simulink model "batterworth_test"  (R2021b)
settings: Solver=VariableStepAuto  StartTime=0.0  StopTime=10.0  RelTol=1e-3
settings Model: Creator=phddk  LastModifiedBy=phddk

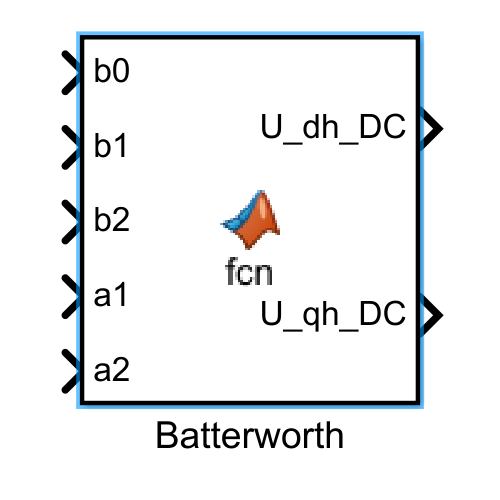
[thumbnail: Simulink's stored preview of the top-level diagram]
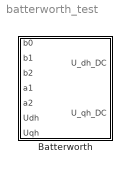
== system batterworth_test ==
  Batterworth : MATLAB Function  TreatAsAtomicUnit=on

== matlab function batterworth_test/Batterworth ==
  data: b0 input; U_dh_DC output; b1 input; b2 input; a1 input; a2 input; U_qh_DC output; Udh input; Uqh input
function [U_dh_DC,U_qh_DC]= fcn(b0,b1,b2,a1,a2,Udh,Uqh)

persistent first_flag
if isempty(first_flag)
    U_dh_DC=0;
    U_qh_DC=0;
    x0=0;
    x1=0;
    x2=0;
    y1=0;
    y2=0;
    x3=0;
    x4=0;
    x5=0;
    y3=0;
    y4=0;
    y0_d=0;
    y0_q=0;

    first_flag=true;
end

x2 = x1;
x1 = x0;
x0 = Udh;

x5 = x4;
x4 = x3;
x3 = Uqh;

y2 = y1;
y1 = y0_d;

y4 = y3;
y3 = y0_q;


U_dh_DC = b0*x0 + b1*x1 + b2*x2 - a1*y1 - a2*y2;
U_qh_DC = b0*x3 + b1*x4 + b2*x5 - a1*y3 - a2*y4;

y0_d = U_dh_DC;
y0_q = U_qh_DC;

end
